simulink model "untitled"  (Simulink 7.4)
settings: Solver=ode45  StartTime=0.0  StopTime=10.0  RelTol=1e-3
libraries: simulink x2
settings Model: Creator=autologin  LastModifiedBy=autologin

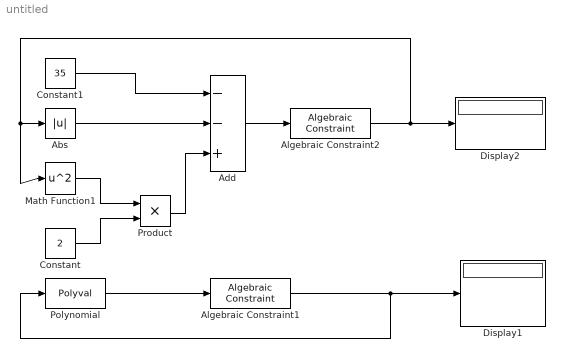
== system untitled ==
  Abs : Abs  OutDataType=fixdt(1, 16)  OutScaling=2^0
  Add : Sum  Inputs=--+  OutDataType=fixdt(1, 16)  OutScaling=2^-10
  Algebraic Constraint1 : simulink/Math Operations/Algebraic Constraint  SystemSampleTime=-1  z0=[-7, -1, 3]
  Algebraic Constraint2 : simulink/Math Operations/Algebraic Constraint  SystemSampleTime=-1  z0=[-4, 4]
  Constant : Constant  Value=2  OutDataType=fixdt(1, 16)  OutScaling=2^0
  Constant1 : Constant  Value=35  OutDataType=fixdt(1, 16)  OutScaling=2^0
  Display1 : Display
  Display2 : Display
  Math Function1 : Math  Operator=square  OutDataType=fixdt(1, 16)  OutScaling=2^0  SaturateOnIntegerOverflow=on
  Polynomial : Polyval  Coefs=[-0.6, -3, 10, 5]
  Product : Product  OutDataType=fixdt(1, 16)  OutScaling=2^0  RndMeth=Zero
  wires:
  Math Function1/1 -> Product/1
  Constant/1 -> Product/2
  Product/1 -> Add/3
  Constant1/1 -> Add/1
  Abs/1 -> Add/2
  Add/1 -> Algebraic Constraint2/1
  Algebraic Constraint2/1 -> Display2/1, Math Function1/1, Abs/1
  Polynomial/1 -> Algebraic Constraint1/1
  Algebraic Constraint1/1 -> Display1/1, Polynomial/1
